simulink model "SF5_5_11_jc0755"  (R2016b)
settings: Solver=VariableStepAuto  StartTime=0.0  StopTime=10.0  RelTol=1e-3
settings Model: Creator=amyyang  LastModifiedBy=amyyang

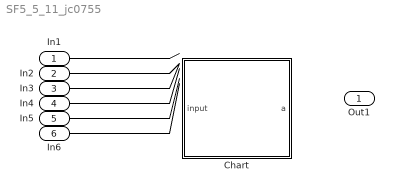
== system SF5_5_11_jc0755 ==
  In1 : Inport
  In2 : Inport  Port=2
  In3 : Inport  Port=3
  In4 : Inport  Port=4
  In5 : Inport  Port=5
  In6 : Inport  Port=6
  Chart : Stateflow chart  TreatAsAtomicUnit=on
  Out1 : Outport
  wires:
  In1/1 -> ?
  In2/1 -> ?
  In3/1 -> ?
  In4/1 -> ?
  In5/1 -> ?
  In6/1 -> ?
  ? -> Out1/1

== stateflow chart SF5_5_11_jc0755/Chart ==
  state A
    en:
    k = 0;
    A -> (junction 2) [order 1]
    (junction 2) -> (junction 3) : {
        |  k++;
        | a = input[k];
        | }
    (junction 3) -> (junction 10) : {
        |  a = input[k++];
        | }
  A -> A [order 1] : { k >= 5}
  data: input input size=6; k local double; a output double
